simulink model "sim4"  (R2022a)
settings: Solver=VariableStepAuto  StartTime=0.0  StopTime=10.0  RelTol=1e-3
libraries: fl_lib x12, dspadpt3 x6, nesl_utility x4, simulink x1
settings Model: Creator=targi  LastModifiedBy=targi

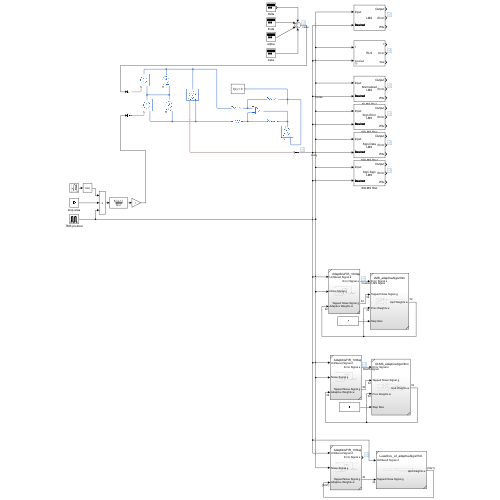
[thumbnail: Simulink's stored preview of the top-level diagram]
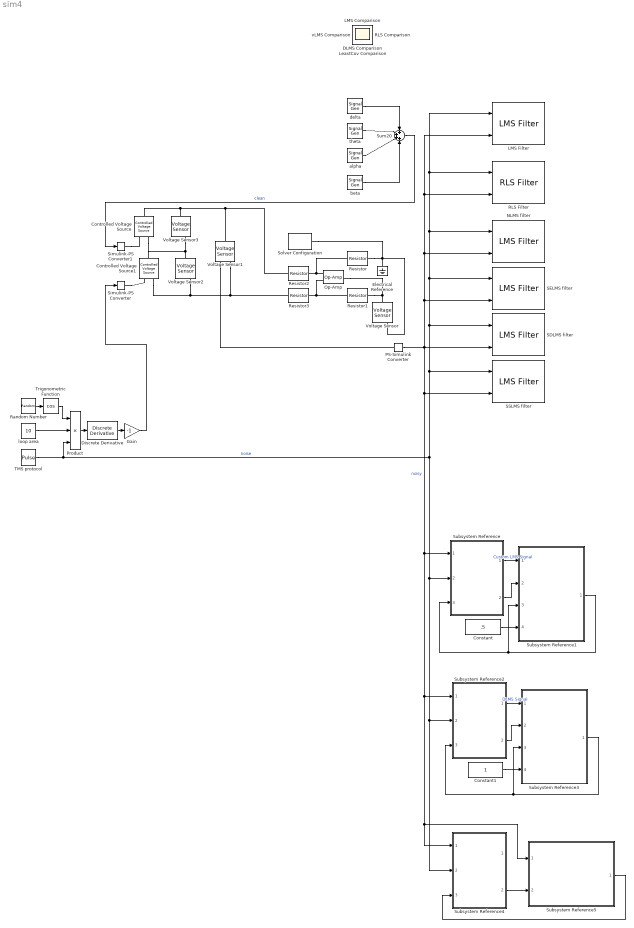
== system sim4 ==
  Constant : Constant  Value=.5
  Constant1 : Constant
  Controlled Voltage Source : fl_lib/Electrical/Electrical Sources/Controlled Voltage Source
      settings: SourceProductBaseCode=PW,SS,VE
  Controlled Voltage Source1 : fl_lib/Electrical/Electrical Sources/Controlled Voltage Source
      settings: SourceProductBaseCode=PW,SS,VE
  Discrete Derivative : simulink/Discrete/Discrete Derivative  gainval=1.0  ICPrevScaledInput=0.0  OutMin=[]  OutMax=[]  OutDataType=fixdt(1, 16)  OutScaling=2^-10  DoSatur=off
  Electrical Reference : fl_lib/Electrical/Electrical Elements/Electrical Reference
      settings: SourceProductBaseCode=PW,SS,VE
  Gain : Gain  Gain=-1
  LMS Filter : dspadpt3/LMS Filter  Algo=LMS  L=32  stepflag=Dialog  mu=0.1  leakage=1.0  ic=0  Adapt=off  resetflag=None  weights=on  addnparflag=off  roundingMode=Floor  overflowMode=off
      settings: SourceProductBaseCode=DS
  NLMS filter : dspadpt3/LMS Filter  Algo=Normalized LMS  L=32  stepflag=Dialog  mu=0.1  leakage=1.0  ic=0  Adapt=off  resetflag=None  weights=on  addnparflag=off  roundingMode=Floor  overflowMode=off
      settings: SourceProductBaseCode=DS
  Op-Amp : fl_lib/Electrical/Electrical Elements/Op-Amp  outI_specify=off  outI_priority=None  outI=0 A  outI_nominal_specify=off  outI_nominal_unit=A  outI_nominal_value=1
      settings: SourceProductBaseCode=PW,SS,VE
  PS-Simulink Converter : nesl_utility/PS-Simulink Converter  PhysicalDomain=network_engine_domain  SubClassName=ps_output  LeftPortType=input  RightPortType=output  PseudoPeriodic=off  Frequencies=[]  VectorFormat=inherit  Unit=inherit  AffineConversion=off
      settings: SourceProductBaseCode=SS,PW,VE
  Product : Product  Inputs=3
  RLS Filter : dspadpt3/RLS Filter  L=32  lambdaflag=Dialog  lambda=1.0  addnparflag=on  ic=0  delta=0.1  Adapt=off  resetflag=None  weights=on
      settings: SourceProductBaseCode=DS
  Random Number : RandomNumber  Variance=.05
  Resistor : fl_lib/Electrical/Electrical Elements/Resistor  R=100 Ohm  i_specify=off  i_priority=None  i=0 A  i_nominal_specify=off  i_nominal_unit=A  i_nominal_value=1  v_specify=off  v_priority=None  v=0 V  v_nominal_specify=off  v_nominal_unit=V  v_nominal_value=1
      settings: SourceProductBaseCode=PW,SS,VE
  Resistor1 : fl_lib/Electrical/Electrical Elements/Resistor  R=100 Ohm  i_specify=off  i_priority=None  i=0 A  i_nominal_specify=off  i_nominal_unit=A  i_nominal_value=1  v_specify=off  v_priority=None  v=0 V  v_nominal_specify=off  v_nominal_unit=V  v_nominal_value=1
      settings: SourceProductBaseCode=PW,SS,VE
  Resistor2 : fl_lib/Electrical/Electrical Elements/Resistor  R=1 Ohm  i_specify=off  i_priority=None  i=0 A  i_nominal_specify=off  i_nominal_unit=A  i_nominal_value=1  v_specify=off  v_priority=None  v=0 V  v_nominal_specify=off  v_nominal_unit=V  v_nominal_value=1
      settings: SourceProductBaseCode=PW,SS,VE
  Resistor3 : fl_lib/Electrical/Electrical Elements/Resistor  R=1 Ohm  i_specify=off  i_priority=None  i=0 A  i_nominal_specify=off  i_nominal_unit=A  i_nominal_value=1  v_specify=off  v_priority=None  v=0 V  v_nominal_specify=off  v_nominal_unit=V  v_nominal_value=1
      settings: SourceProductBaseCode=PW,SS,VE
  SDLMS filter : dspadpt3/LMS Filter  Algo=Sign-Data LMS  L=32  stepflag=Dialog  mu=0.1  leakage=1.0  ic=0  Adapt=off  resetflag=None  weights=on  addnparflag=off  roundingMode=Floor  overflowMode=off
      settings: SourceProductBaseCode=DS
  SELMS filter : dspadpt3/LMS Filter  Algo=Sign-Error LMS  L=32  stepflag=Dialog  mu=0.01  leakage=1.0  ic=0  Adapt=off  resetflag=None  weights=on  addnparflag=off  roundingMode=Floor  overflowMode=off
      settings: SourceProductBaseCode=DS
  SSLMS filter : dspadpt3/LMS Filter  Algo=Sign-Sign LMS  L=32  stepflag=Dialog  mu=0.01  leakage=1.0  ic=0  Adapt=off  resetflag=None  weights=on  addnparflag=off  roundingMode=Floor  overflowMode=off
      settings: SourceProductBaseCode=DS
  Simulink-PS Converter : nesl_utility/Simulink-PS Converter  PhysicalDomain=network_engine_domain  SubClassName=ps_input  LeftPortType=input  RightPortType=output  PseudoPeriodic=off  Frequencies=[]  NoiseDistribution=none  NoiseParameters=[]  Unit=1  AffineConversion=off  FilteringAndDerivatives=provide  SimscapeFilterOrder=1  InputFilterTimeConstant=0.001  UdotUserProvided=0
      settings: SourceProductBaseCode=SS,PW,VE
  Simulink-PS Converter1 : nesl_utility/Simulink-PS Converter  PhysicalDomain=network_engine_domain  SubClassName=ps_input  LeftPortType=input  RightPortType=output  PseudoPeriodic=off  Frequencies=[]  NoiseDistribution=none  NoiseParameters=[]  Unit=1  AffineConversion=off  FilteringAndDerivatives=provide  SimscapeFilterOrder=1  InputFilterTimeConstant=0.001  UdotUserProvided=0
      settings: SourceProductBaseCode=SS,PW,VE
  Solver Configuration : nesl_utility/Solver Configuration  PhysicalDomain=network_engine_domain  SubClassName=solver  LeftPortType=input  RightPortType=generic  Tones=[]  Harmonics=[]  SimulateNoise=off  Profile=off  UseLocalSampling=off  EnableSwitchedLinearOptims=on  FrequencyDomain=off  UseCCode=off  RelTol=0.001  AbsTol=0.001  MinStep=1e-09  ToWorkspace=off  RevertToSquareIcSolve=off  NumHomotopyIterations=100  PhasorMode=off  PhasorModeNumHarmonics=1  IndexReductionMethod=DerivativeReplacement  DoDC=off  ResidualTolerance=1e-09  UseLocalSolver=off  LocalSolverChoice=NE_BACKWARD_EULER_ADVANCER  LocalSolverSampleTime=0.001  DoFixedCost=off  MaxNonlinIter=3  MaxModeIter=2  ComputeImpulses=off  ImpulseIterations=2  LinearAlgebra=auto  LinearAlgebraNumThread=0  EquationFormulation=NE_TIME_EF  DelaysMemoryBudget=1024  AutomaticFiltering=on  FilteringTimeConstant=0.001  PartitionStorageMethod=AS_NEEDED  PartitionMemoryBudget=1024  PartitionMethod=ROBUST
      settings: SourceProductBaseCode=SS,PW,VE
  Subsystem Reference : Subsystem  ReferencedSubsystem=AdaptibleFIR_100taps
  Subsystem Reference1 : Subsystem  ReferencedSubsystem=LMS_adaptiveAlgorithm
  Subsystem Reference2 : Subsystem  ReferencedSubsystem=AdaptibleFIR_100taps
  Subsystem Reference3 : Subsystem  ReferencedSubsystem=DLMS_adaptiveAlgorithm
  Subsystem Reference4 : Subsystem  ReferencedSubsystem=AdaptibleFIR_100taps
  Subsystem Reference5 : Subsystem  ReferencedSubsystem=LeastCov_v2_adaptiveAlgorithm
  Sum20 : Sum  Inputs=++++
  TMS protocol : DiscretePulseGenerator  PulseType=Time based  Period=.1  PulseWidth=5
  Trigonometric Function : Trigonometry  Operator=cos
  Voltage Sensor{,1..3} (4 alike) : fl_lib/Electrical/Electrical Sensors/Voltage Sensor
      settings: SourceProductBaseCode=PW,SS,VE
  alpha : SignalGenerator  Amplitude=.002  Frequency=10
  beta : SignalGenerator  Amplitude=.001  Frequency=22
  delta : SignalGenerator  Amplitude=.004  Frequency=2
  loop area : Constant  Value=10
  theta : SignalGenerator  Amplitude=.003  Frequency=6
  DLMS Comparison : Scope
  LMS Comparison : Scope
  LeastCov Comparison : Scope
  RLS Comparison : Scope
  vLMS Comparison : Scope
  wires:
  delta/1 -> Sum20/1
  TMS protocol/1 -> Product/3, Subsystem Reference4/2, Subsystem Reference2/2, Subsystem Reference/2, RLS Filter/1, LMS Filter/1, NLMS filter/1, SELMS filter/1, SDLMS filter/1, SSLMS filter/1  "noise"
  theta/1 -> Sum20/2
  Sum20/1 -> Simulink-PS Converter1/1  "clean"
  beta/1 -> Sum20/4
  alpha/1 -> Sum20/3
  PS-Simulink Converter/1 -> Subsystem Reference5/1, Subsystem Reference4/1, Subsystem Reference2/1, Subsystem Reference/1, SSLMS filter/2, LMS Filter/2, RLS Filter/2, NLMS filter/2, SELMS filter/2, SDLMS filter/2  "noisy"
  Subsystem Reference/1 -> Subsystem Reference1/1  "Custom LMS Signal"
  Subsystem Reference/2 -> Subsystem Reference1/2
  Subsystem Reference1/1 -> Subsystem Reference1/3, Subsystem Reference/3
  Constant/1 -> Subsystem Reference1/4
  Constant1/1 -> Subsystem Reference3/4
  Subsystem Reference2/2 -> Subsystem Reference3/2
  Subsystem Reference2/1 -> Subsystem Reference3/1  "DLMS Signal"
  Subsystem Reference3/1 -> Subsystem Reference3/3, Subsystem Reference2/3
  loop area/1 -> Product/2
  Random Number/1 -> Trigonometric Function/1
  Trigonometric Function/1 -> Product/1
  Product/1 -> Discrete Derivative/1
  Discrete Derivative/1 -> Gain/1
  Gain/1 -> Simulink-PS Converter/1
  Subsystem Reference4/2 -> Subsystem Reference5/2
  Subsystem Reference5/1 -> Subsystem Reference4/3
  connections:
  Resistor2/RConn1 -- Resistor/LConn1 -- Op-Amp/LConn1
  Resistor1/LConn1 -- Op-Amp/LConn2 -- Resistor3/RConn1
  Op-Amp/RConn1 -- Resistor1/RConn1 -- Voltage Sensor/LConn1
  Resistor/RConn1 -- Solver Configuration/RConn1 -- Electrical Reference/LConn1 -- Voltage Sensor/RConn2
  Resistor2/LConn1 -- Controlled Voltage Source/LConn1 -- Voltage Sensor3/LConn1 -- Voltage Sensor1/LConn1
  Voltage Sensor3/RConn2 -- Controlled Voltage Source/RConn2 -- Controlled Voltage Source1/LConn1 -- Voltage Sensor2/LConn1
  Voltage Sensor1/RConn2 -- Controlled Voltage Source1/RConn2 -- Voltage Sensor2/RConn2 -- Resistor3/LConn1
  Simulink-PS Converter/RConn1 -- Controlled Voltage Source1/RConn1
  Simulink-PS Converter1/RConn1 -- Controlled Voltage Source/RConn1
  Voltage Sensor1/RConn1 -- PS-Simulink Converter/LConn1
